simulink model "IntegratedDepthWheel"  (R2024a)
settings: Solver=VariableStepAuto  StartTime=0.0  StopTime=100  FixedStep=0.01  MaxStep=0.01  RelTol=1e-6
model workspace (MAT data in the model file):
  E_A = 10000000
  L0_init = 100
  Lambda_eff_g = 7.85
  r_wheel = 0.0508
  rho_mud = 1200
  w_tool_g = 2943
libraries: fl_lib x24, nesl_utility x9, sdl_lib x1
settings Model: Creator=Youssef  LastModifiedBy=Youssef

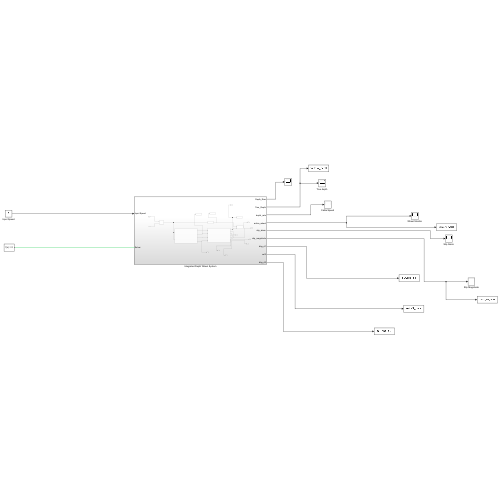
[thumbnail: Simulink's stored preview of the top-level diagram]
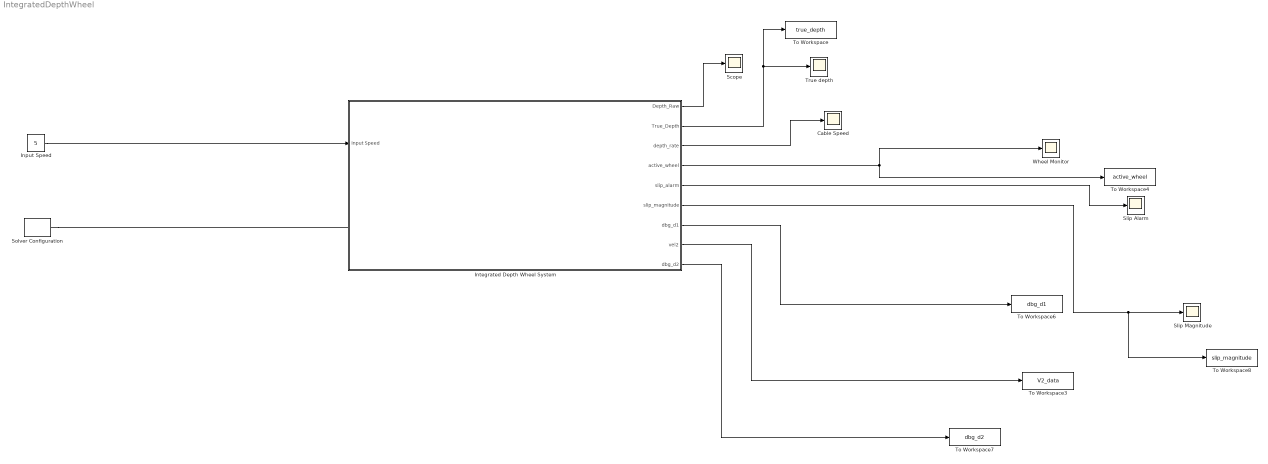
== system IntegratedDepthWheel ==
  Cable Speed : Scope
  Input Speed : Constant  Value=5
  Integrated Depth Wheel System : Subsystem
  Scope : Scope
  Slip Alarm : Scope
  Slip Magnitude : Scope
  Solver Configuration : nesl_utility/Solver Configuration  PhysicalDomain=network_engine_domain  SubClassName=solver  LeftPortType=input  RightPortType=generic  Tones=[]  Harmonics=[]  SimulateNoise=off  Profile=off  UseLocalSampling=off  EnableSwitchedLinearOptims=on  FrequencyDomain=off  UseCCode=off  RelTol=0.001  AbsTol=0.001  MinStep=1e-09  ToWorkspace=off  RevertToSquareIcSolve=off  NumHomotopyIterations=100  PhasorMode=off  PhasorModeNumHarmonics=1  ConsistencySolver=NEWTON_XTOL_AFTER_FTOL  IndexReductionMethod=DerivativeReplacement  DoDC=off  ResidualTolerance=1e-09  ConsistencyTolSource=GLOBAL  ConsistencyAbsTol=0.001  ConsistencyRelTol=0.001  ConsistencyTolFactor=0.001  UseLocalSolver=on  LocalSolverChoice=NE_TRAPEZOIDAL_ADVANCER  ResolveIndetEquations=on  FunctionEvalNumThread=1  LocalSolverSampleTime=0.01  DoFixedCost=on  MaxNonlinIter=3  MaxModeIter=2  ComputeImpulses=off  ImpulseIterations=2  LinearAlgebra=auto  LinearAlgebraNumThread=0  EquationFormulation=NE_TIME_EF  DelaysMemoryBudget=1024  AutomaticFiltering=on  FilteringTimeConstant=0.001  PartitionStorageMethod=AS_NEEDED  PartitionMemoryBudget=1024  PartitionMethod=ROBUST  MultibodyUseLocalSolver=off  MultibodyLocalSolverChoice=ODE1  MultibodyLocalSolverSampleTime=0.001
  To Workspace : ToWorkspace  VariableName=true_depth  SaveFormat=Timeseries  SampleTime=-1
  To Workspace3 : ToWorkspace  VariableName=V2_data  SaveFormat=Timeseries  SampleTime=-1
  To Workspace4 : ToWorkspace  VariableName=active_wheel  SaveFormat=Timeseries  SampleTime=-1
  To Workspace6 : ToWorkspace  VariableName=dbg_d1  SaveFormat=Timeseries  SampleTime=-1
  To Workspace7 : ToWorkspace  VariableName=dbg_d2  SaveFormat=Timeseries  SampleTime=-1
  To Workspace8 : ToWorkspace  VariableName=slip_magnitude  SaveFormat=Timeseries  SampleTime=-1
  True depth : Scope
  Wheel Monitor : Scope
  wires:
  Integrated Depth Wheel System/4(active_wheel) -> Wheel Monitor/1, To Workspace4/1
  Integrated Depth Wheel System/6(slip_magnitude) -> To Workspace8/1, Slip Magnitude/1
  Integrated Depth Wheel System/2(True_Depth) -> To Workspace/1, True depth/1
  Input Speed/1 -> Integrated Depth Wheel System/1(Input Speed)
  Integrated Depth Wheel System/1(Depth_Raw) -> Scope/1
  Integrated Depth Wheel System/3(depth_rate) -> Cable Speed/1
  Integrated Depth Wheel System/5(slip_alarm) -> Slip Alarm/1
  Integrated Depth Wheel System/7(dbg_d1) -> To Workspace6/1
  Integrated Depth Wheel System/8(vel2) -> To Workspace3/1
  Integrated Depth Wheel System/9(dbg_d2) -> To Workspace7/1
  connections:
  Solver Configuration/RConn1 -- Integrated Depth Wheel System/LConn1

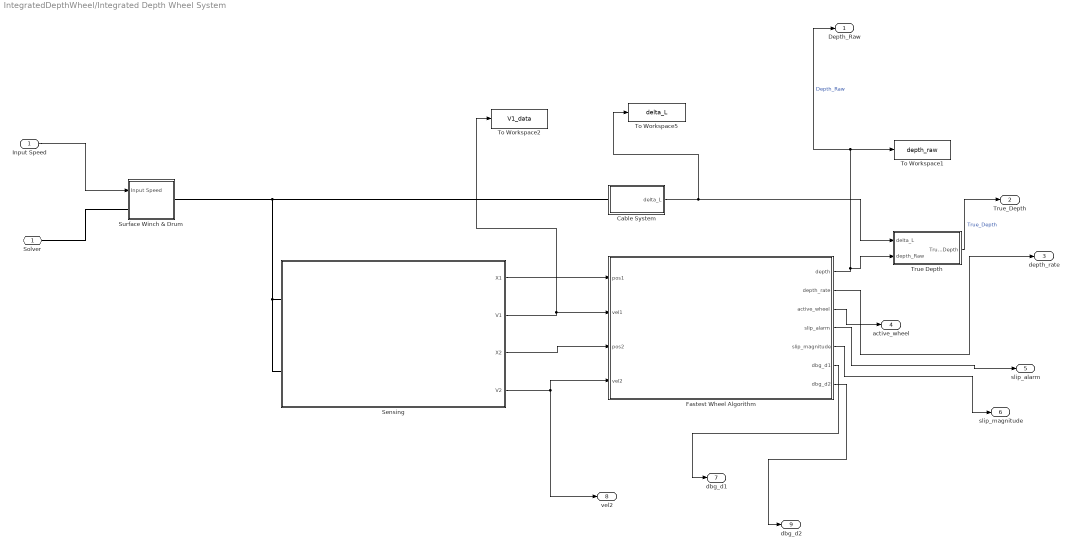
== system IntegratedDepthWheel/Integrated Depth Wheel System ==
  Input Speed : Inport
  Cable System : Subsystem
  Fastest Wheel Algorithm : MATLAB Function  TreatAsAtomicUnit=on  SystemSampleTime=0.01
  Sensing : Subsystem
  Surface Winch & Drum : Subsystem
  To Workspace1 : ToWorkspace  VariableName=depth_raw  SaveFormat=Timeseries  SampleTime=-1
  To Workspace2 : ToWorkspace  VariableName=V1_data  SaveFormat=Timeseries  SampleTime=-1
  To Workspace5 : ToWorkspace  VariableName=delta_L  SaveFormat=Timeseries  SampleTime=-1
  True Depth : Subsystem
  Solver : PMIOPort  Side=Left
  Depth_Raw : Outport
  True_Depth : Outport  Port=2
  depth_rate : Outport  Port=3
  active_wheel : Outport  Port=4
  slip_alarm : Outport  Port=5
  slip_magnitude : Outport  Port=6
  dbg_d1 : Outport  Port=7
  vel2 : Outport  Port=8
  dbg_d2 : Outport  Port=9
  wires:
  Cable System/1(delta_L) -> To Workspace5/1, True Depth/1(delta_L)
  Fastest Wheel Algorithm/1(depth) -> Depth_Raw/1, To Workspace1/1, True Depth/2(depth_Raw)  "Depth_Raw"
  Sensing/2(V1) -> To Workspace2/1, Fastest Wheel Algorithm/2(vel1)
  Sensing/4(V2) -> vel2/1, Fastest Wheel Algorithm/4(vel2)
  Sensing/3(X2) -> Fastest Wheel Algorithm/3(pos2)
  Input Speed/1 -> Surface Winch & Drum/1(Input Speed)
  Sensing/1(X1) -> Fastest Wheel Algorithm/1(pos1)
  True Depth/1(True Depth) -> True_Depth/1  "True_Depth"
  Fastest Wheel Algorithm/2(depth_rate) -> depth_rate/1
  Fastest Wheel Algorithm/5(slip_magnitude) -> slip_magnitude/1
  Fastest Wheel Algorithm/6(dbg_d1) -> dbg_d1/1
  Fastest Wheel Algorithm/4(slip_alarm) -> slip_alarm/1
  Fastest Wheel Algorithm/7(dbg_d2) -> dbg_d2/1
  Fastest Wheel Algorithm/3(active_wheel) -> active_wheel/1
  connections:
  Surface Winch & Drum/RConn1 -- Sensing/LConn2 -- Sensing/LConn1 -- Cable System/LConn1
  Solver/RConn1 -- Surface Winch & Drum/LConn1

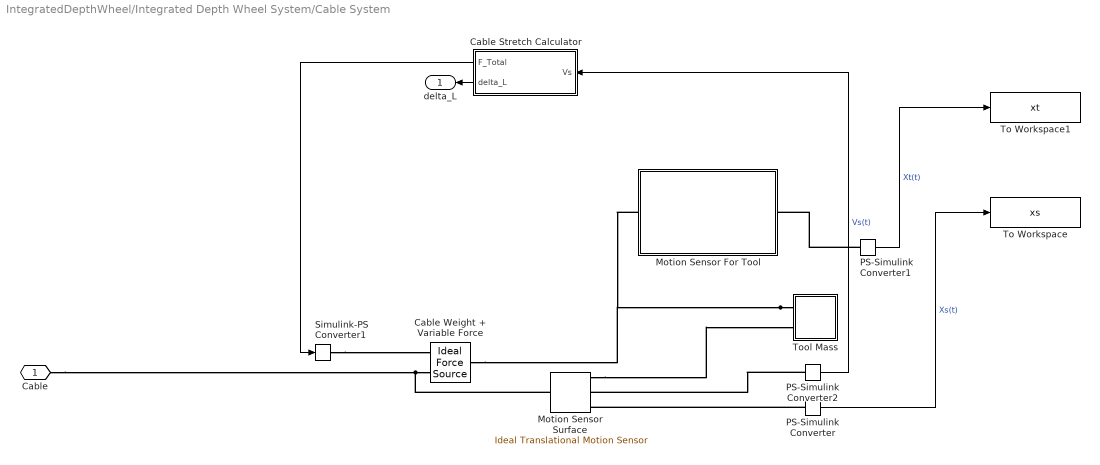
== system IntegratedDepthWheel/Integrated Depth Wheel System/Cable System ==
  " Cable Stretch Calculator" : Subsystem
  Cable Weight + Variable Force : fl_lib/Mechanical/Mechanical Sources/Ideal Force Source
  Motion Sensor For Tool : Subsystem
  Motion Sensor Surface : fl_lib/Mechanical/Mechanical Sensors/Ideal Translational Motion Sensor  reference=foundation.enum.MeasurementReference.difference  acceleration_port=false  velocity_port=true  position_port=true  offset=0 m
  PS-Simulink Converter : nesl_utility/PS-Simulink Converter  PhysicalDomain=network_engine_domain  SubClassName=ps_output  LeftPortType=input  RightPortType=output  PseudoPeriodic=off  Frequencies=[]  VectorFormat=inherit  Unit=inherit  AffineConversion=off
  PS-Simulink Converter1 : nesl_utility/PS-Simulink Converter  PhysicalDomain=network_engine_domain  SubClassName=ps_output  LeftPortType=input  RightPortType=output  PseudoPeriodic=off  Frequencies=[]  VectorFormat=inherit  Unit=inherit  AffineConversion=off
  PS-Simulink Converter2 : nesl_utility/PS-Simulink Converter  PhysicalDomain=network_engine_domain  SubClassName=ps_output  LeftPortType=input  RightPortType=output  PseudoPeriodic=off  Frequencies=[]  VectorFormat=inherit  Unit=inherit  AffineConversion=off
  Simulink-PS Converter1 : nesl_utility/Simulink-PS Converter  PhysicalDomain=network_engine_domain  SubClassName=ps_input  LeftPortType=input  RightPortType=output  PseudoPeriodic=off  Frequencies=[]  NoiseDistribution=none  NoiseParameters=[]  Unit=1  AffineConversion=off  FilteringAndDerivatives=filter  SimscapeFilterOrder=1  InputFilterTimeConstant=0.01  UdotUserProvided=0
  To Workspace : ToWorkspace  VariableName=xs  SaveFormat=Timeseries  SampleTime=-1
  To Workspace1 : ToWorkspace  VariableName=xt  SaveFormat=Timeseries  SampleTime=-1
  Tool Mass : Subsystem
  Cable : PMIOPort  Side=Left
  delta_L : Outport
  wires:
  " Cable Stretch Calculator"/2(delta_L) -> delta_L/1
  PS-Simulink Converter1/1 -> To Workspace1/1  "Xt(t)"
  " Cable Stretch Calculator"/1(F_Total) -> Simulink-PS Converter1/1
  PS-Simulink Converter/1 -> To Workspace/1  "Xs(t)"
  PS-Simulink Converter2/1 -> " Cable Stretch Calculator"/1(Vs)  "Vs(t)"
  connections:
  PS-Simulink Converter1/LConn1 -- Motion Sensor For Tool/RConn1
  Simulink-PS Converter1/RConn1 -- Cable Weight + Variable Force/RConn1
  Motion Sensor Surface/RConn1 -- Tool Mass/LConn2
  PS-Simulink Converter/LConn1 -- Motion Sensor Surface/RConn3
  Motion Sensor Surface/LConn1 -- Cable/RConn1 -- Cable Weight + Variable Force/RConn2
  Tool Mass/LConn1 -- Cable Weight + Variable Force/LConn1 -- Motion Sensor For Tool/LConn1
  PS-Simulink Converter2/LConn1 -- Motion Sensor Surface/RConn2

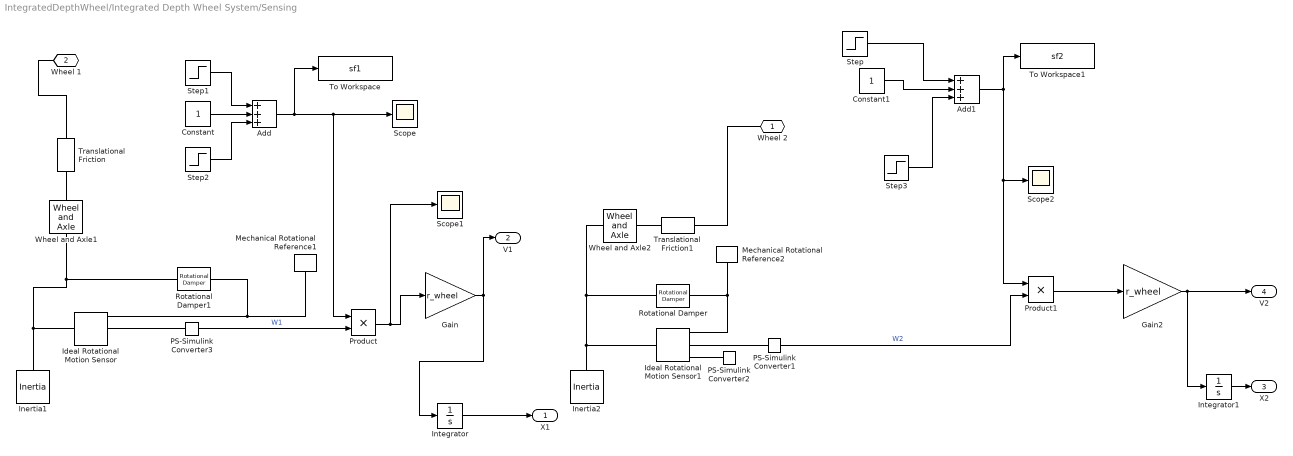
== system IntegratedDepthWheel/Integrated Depth Wheel System/Sensing ==
  Add : Sum  Inputs=+++
  Add1 : Sum  Inputs=+++
  Constant : Constant
  Constant1 : Constant
  Gain : Gain  Gain=r_wheel
  Gain2 : Gain  Gain=r_wheel
  Ideal Rotational Motion Sensor : fl_lib/Mechanical/Mechanical Sensors/Ideal Rotational Motion Sensor  reference=foundation.enum.MeasurementReference.difference  acceleration_port=false  velocity_port=true  position_port=true  wrap_angle=false  offset=0 rad
  Ideal Rotational Motion Sensor1 : fl_lib/Mechanical/Mechanical Sensors/Ideal Rotational Motion Sensor  reference=foundation.enum.MeasurementReference.difference  acceleration_port=false  velocity_port=true  position_port=true  wrap_angle=false  offset=0 rad
  Inertia1 : fl_lib/Mechanical/Rotational Elements/Inertia  inertia=0.02 kg*m^2  num_ports=foundation.enum.numPorts2.one  w_specify=off  w_priority=High  w=0 rad/s  w_nominal_specify=off  w_nominal_value=1  w_nominal_unit=rad/s  t_specify=off  t_priority=None  t=0 N*m  t_nominal_specify=off  t_nominal_value=1  t_nominal_unit=N*m
  Inertia2 : fl_lib/Mechanical/Rotational Elements/Inertia  inertia=0.02 kg*m^2  num_ports=foundation.enum.numPorts2.one  w_specify=off  w_priority=High  w=0 rad/s  w_nominal_specify=off  w_nominal_value=1  w_nominal_unit=rad/s  t_specify=off  t_priority=None  t=0 N*m  t_nominal_specify=off  t_nominal_value=1  t_nominal_unit=N*m
  Integrator : Integrator
  Integrator1 : Integrator
  Mechanical Rotational Reference1 : fl_lib/Mechanical/Rotational Elements/Mechanical Rotational Reference
  Mechanical Rotational Reference2 : fl_lib/Mechanical/Rotational Elements/Mechanical Rotational Reference
  PS-Simulink Converter1 : nesl_utility/PS-Simulink Converter  PhysicalDomain=network_engine_domain  SubClassName=ps_output  LeftPortType=input  RightPortType=output  PseudoPeriodic=off  Frequencies=[]  VectorFormat=inherit  Unit=inherit  AffineConversion=off
  PS-Simulink Converter2 : nesl_utility/PS-Simulink Converter  PhysicalDomain=network_engine_domain  SubClassName=ps_output  LeftPortType=input  RightPortType=output  PseudoPeriodic=off  Frequencies=[]  VectorFormat=inherit  Unit=inherit  AffineConversion=off
  PS-Simulink Converter3 : nesl_utility/PS-Simulink Converter  PhysicalDomain=network_engine_domain  SubClassName=ps_output  LeftPortType=input  RightPortType=output  PseudoPeriodic=off  Frequencies=[]  VectorFormat=inherit  Unit=inherit  AffineConversion=off
  Product : Product
  Product1 : Product
  Rotational Damper : fl_lib/Mechanical/Rotational Elements/Rotational Damper  D=0.001 N*m*s/rad  w_specify=off  w_priority=None  w=0 rad/s  w_nominal_specify=off  w_nominal_value=1  w_nominal_unit=rad/s  t_specify=off  t_priority=None  t=0 N*m  t_nominal_specify=off  t_nominal_value=1  t_nominal_unit=N*m
  Rotational Damper1 : fl_lib/Mechanical/Rotational Elements/Rotational Damper  D=0.001 N*m*s/rad  w_specify=off  w_priority=None  w=0 rad/s  w_nominal_specify=off  w_nominal_value=1  w_nominal_unit=rad/s  t_specify=off  t_priority=None  t=0 N*m  t_nominal_specify=off  t_nominal_value=1  t_nominal_unit=N*m
  Scope : Scope
  Scope1 : Scope
  Scope2 : Scope
  Step : Step  Time=55  After=-0.4  SampleTime=0
  Step1 : Step  Time=35  After=-0.2  SampleTime=0
  Step2 : Step  Time=50  After=0.2  SampleTime=0
  Step3 : Step  Time=70  After=0.4  SampleTime=0
  To Workspace : ToWorkspace  VariableName=sf1  SaveFormat=Timeseries  SampleTime=-1
  To Workspace1 : ToWorkspace  VariableName=sf2  SaveFormat=Timeseries  SampleTime=-1
  Translational Friction : fl_lib/Mechanical/Translational Elements/Translational Friction  brkwy_frc=100 N  brkwy_vel=0.1 m/s  Col_frc=20 N  visc_coef=100 N*s/m  v_specify=off  v_priority=None  v=0 m/s  v_nominal_specify=off  v_nominal_value=1  v_nominal_unit=m/s  f_specify=off  f_priority=None  f=0 N  f_nominal_specify=off  f_nominal_value=1  f_nominal_unit=N
      settings: InternalSimscapePortConfiguration="{\"Bottom\":[],\"Left\":[{\"id\":\"R\",\"label\":\"R\",\"type\":\"foundation.mechanical.translational.translational\"}],\"Right\":[{\"id\":\"C\",\"label\":\"C\",\"type\":\"foundation.mechanical.translational.translational\"}],\"Top\":[]}"
  Translational Friction1 : fl_lib/Mechanical/Translational Elements/Translational Friction  brkwy_frc=90 N  brkwy_vel=0.1 m/s  Col_frc=20 N  visc_coef=100 N*s/m  v_specify=off  v_priority=None  v=0 m/s  v_nominal_specify=off  v_nominal_value=1  v_nominal_unit=m/s  f_specify=off  f_priority=None  f=0 N  f_nominal_specify=off  f_nominal_value=1  f_nominal_unit=N
      settings: InternalSimscapePortConfiguration="{\"Bottom\":[],\"Left\":[{\"id\":\"R\",\"label\":\"R\",\"type\":\"foundation.mechanical.translational.translational\"}],\"Right\":[{\"id\":\"C\",\"label\":\"C\",\"type\":\"foundation.mechanical.translational.translational\"}],\"Top\":[]}"
  Wheel and Axle1 : fl_lib/Mechanical/Mechanisms/Wheel and Axle  R=r_wheel m  or=1  t_specify=off  t_priority=None  t=0 N*m  t_nominal_specify=off  t_nominal_value=1  t_nominal_unit=N*m  f_specify=off  f_priority=None  f=0 N  f_nominal_specify=off  f_nominal_value=1  f_nominal_unit=N
  Wheel and Axle2 : fl_lib/Mechanical/Mechanisms/Wheel and Axle  R=r_wheel m  or=1  t_specify=off  t_priority=None  t=0 N*m  t_nominal_specify=off  t_nominal_value=1  t_nominal_unit=N*m  f_specify=off  f_priority=None  f=0 N  f_nominal_specify=off  f_nominal_value=1  f_nominal_unit=N
  Wheel 2 : PMIOPort  Side=Left
  Wheel 1 : PMIOPort  Port=2  Side=Left
  X1 : Outport
  V1 : Outport  Port=2
  X2 : Outport  Port=3
  V2 : Outport  Port=4
  wires:
  PS-Simulink Converter3/1 -> Product/2  "W1"
  Gain/1 -> Integrator/1, V1/1
  Gain2/1 -> V2/1, Integrator1/1
  Add/1 -> To Workspace/1, Product/1, Scope/1
  Product/1 -> Scope1/1, Gain/1
  Product1/1 -> Gain2/1
  PS-Simulink Converter1/1 -> Product1/2  "W2"
  Integrator/1 -> X1/1
  Integrator1/1 -> X2/1
  Add1/1 -> To Workspace1/1, Scope2/1, Product1/1
  Step1/1 -> Add/1
  Step2/1 -> Add/3
  Constant/1 -> Add/2
  Step/1 -> Add1/1
  Constant1/1 -> Add1/2
  Step3/1 -> Add1/3
  connections:
  Inertia1/LConn1 -- Ideal Rotational Motion Sensor/LConn1 -- Rotational Damper1/LConn1 -- Wheel and Axle1/LConn1
  Inertia2/LConn1 -- Ideal Rotational Motion Sensor1/LConn1 -- Wheel and Axle2/LConn1 -- Rotational Damper/LConn1
  Translational Friction1/LConn1 -- Wheel and Axle2/RConn1
  Ideal Rotational Motion Sensor/RConn1 -- Rotational Damper1/RConn1 -- Mechanical Rotational Reference1/LConn1
  Wheel and Axle1/RConn1 -- Translational Friction/LConn1
  Translational Friction/RConn1 -- Wheel 1/RConn1
  Translational Friction1/RConn1 -- Wheel 2/RConn1
  PS-Simulink Converter3/LConn1 -- Ideal Rotational Motion Sensor/RConn2
  Ideal Rotational Motion Sensor1/RConn1 -- Mechanical Rotational Reference2/LConn1 -- Rotational Damper/RConn1
  PS-Simulink Converter1/LConn1 -- Ideal Rotational Motion Sensor1/RConn2
  PS-Simulink Converter2/LConn1 -- Ideal Rotational Motion Sensor1/RConn3

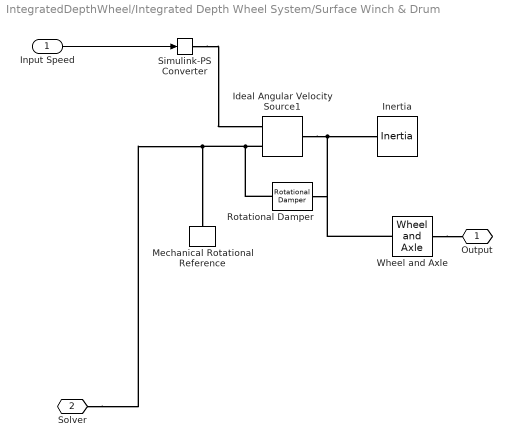
== system IntegratedDepthWheel/Integrated Depth Wheel System/Surface Winch & Drum ==
  Input Speed : Inport
  Ideal Angular Velocity Source1 : fl_lib/Mechanical/Mechanical Sources/Ideal Angular Velocity Source
  Inertia : fl_lib/Mechanical/Rotational Elements/Inertia  inertia=500 kg*m^2  num_ports=foundation.enum.numPorts2.one  w_specify=off  w_priority=High  w=0 rad/s  w_nominal_specify=off  w_nominal_value=1  w_nominal_unit=rad/s  t_specify=off  t_priority=None  t=0 N*m  t_nominal_specify=off  t_nominal_value=1  t_nominal_unit=N*m
  Mechanical Rotational Reference : fl_lib/Mechanical/Rotational Elements/Mechanical Rotational Reference
  Rotational Damper : fl_lib/Mechanical/Rotational Elements/Rotational Damper  D=0.001 N*m*s/rad  w_specify=off  w_priority=None  w=0 rad/s  w_nominal_specify=off  w_nominal_value=1  w_nominal_unit=rad/s  t_specify=off  t_priority=None  t=0 N*m  t_nominal_specify=off  t_nominal_value=1  t_nominal_unit=N*m
  Simulink-PS Converter : nesl_utility/Simulink-PS Converter  PhysicalDomain=network_engine_domain  SubClassName=ps_input  LeftPortType=input  RightPortType=output  PseudoPeriodic=off  Frequencies=[]  NoiseDistribution=none  NoiseParameters=[]  Unit=1  AffineConversion=off  FilteringAndDerivatives=provide  SimscapeFilterOrder=1  InputFilterTimeConstant=0.001  UdotUserProvided=0
  Wheel and Axle : fl_lib/Mechanical/Mechanisms/Wheel and Axle  R=0.4 m  or=1  t_specify=off  t_priority=None  t=0 N*m  t_nominal_specify=off  t_nominal_value=1  t_nominal_unit=N*m  f_specify=off  f_priority=None  f=0 N  f_nominal_specify=off  f_nominal_value=1  f_nominal_unit=N
  Output : PMIOPort  Side=Right
  Solver : PMIOPort  Port=2  Side=Left
  wires:
  Input Speed/1 -> Simulink-PS Converter/1
  connections:
  Ideal Angular Velocity Source1/RConn2 -- Rotational Damper/RConn1 -- Solver/RConn1 -- Mechanical Rotational Reference/LConn1
  Ideal Angular Velocity Source1/LConn1 -- Wheel and Axle/LConn1 -- Rotational Damper/LConn1 -- Inertia/LConn1
  Simulink-PS Converter/RConn1 -- Ideal Angular Velocity Source1/RConn1
  Wheel and Axle/RConn1 -- Output/RConn1

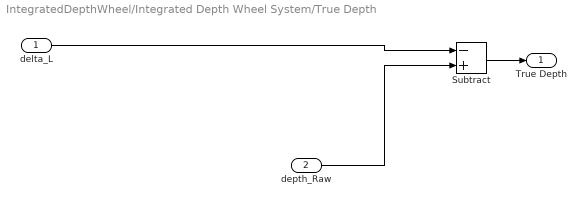
== system IntegratedDepthWheel/Integrated Depth Wheel System/True Depth ==
  delta_L : Inport
  depth_Raw : Inport  Port=2
  Subtract : Sum  Inputs=-+
  True Depth : Outport
  wires:
  delta_L/1 -> Subtract/1
  depth_Raw/1 -> Subtract/2
  Subtract/1 -> True Depth/1

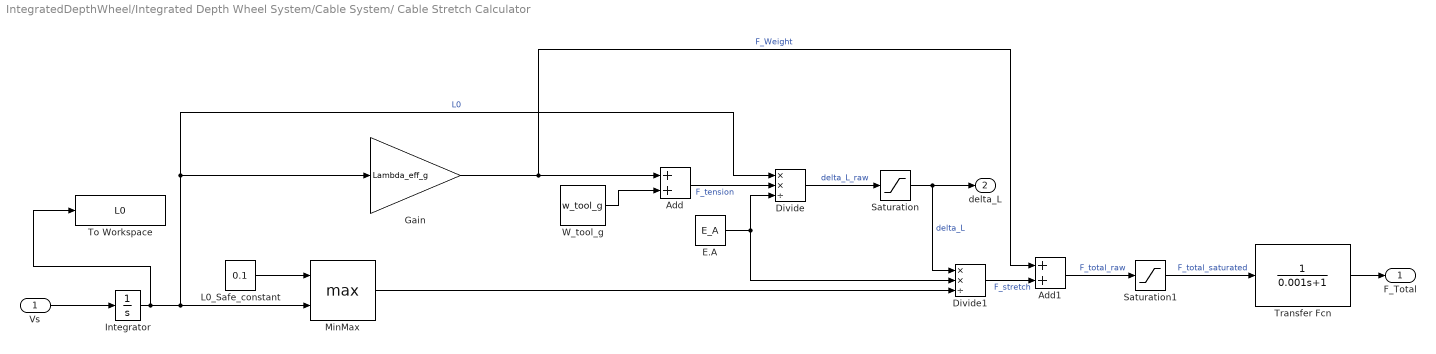
== system IntegratedDepthWheel/Integrated Depth Wheel System/Cable System/ Cable Stretch Calculator ==
  Vs : Inport
  Add : Sum
  Add1 : Sum
  Divide : Product  Inputs=**/
  Divide1 : Product  Inputs=**/
  E.A : Constant  Value=E_A
  Gain : Gain  Gain=Lambda_eff_g
  Integrator : Integrator  InitialCondition=L0_init
  L0_Safe_constant : Constant  Value=0.1
  MinMax : MinMax  Function=max  Inputs=2
  Saturation : Saturate  UpperLimit=inf  LowerLimit=0
  Saturation1 : Saturate  UpperLimit=50000  LowerLimit=0
  To Workspace : ToWorkspace  VariableName=L0  SaveFormat=Timeseries  SampleTime=-1
  Transfer Fcn : TransferFcn  Denominator=[0.001 1]
  W_tool_g : Constant  Value=w_tool_g
  F_Total : Outport
  delta_L : Outport  Port=2
  wires:
  Vs/1 -> Integrator/1
  Integrator/1 -> To Workspace/1, Divide/1, Gain/1, MinMax/2  "L0"
  L0_Safe_constant/1 -> MinMax/1
  Gain/1 -> Add1/1, Add/1  "F_Weight"
  W_tool_g/1 -> Add/2
  Add/1 -> Divide/2  "F_tension"
  E.A/1 -> Divide1/2, Divide/3
  Divide/1 -> Saturation/1  "delta_L_raw"
  Saturation/1 -> Divide1/1, delta_L/1  "delta_L"
  MinMax/1 -> Divide1/3
  Divide1/1 -> Add1/2  "F_stretch"
  Add1/1 -> Saturation1/1  "F_total_raw"
  Saturation1/1 -> Transfer Fcn/1  "F_total_saturated"
  Transfer Fcn/1 -> F_Total/1

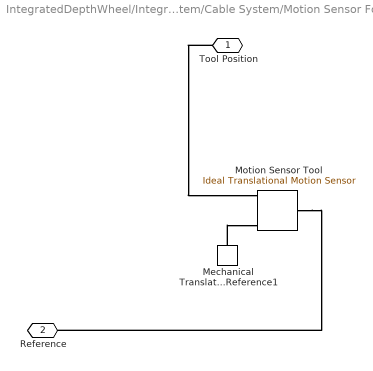
== system IntegratedDepthWheel/Integrated Depth Wheel System/Cable System/Motion Sensor For Tool ==
  Mechanical Translational Reference1 : fl_lib/Mechanical/Translational Elements/Mechanical Translational Reference
  Motion Sensor Tool : fl_lib/Mechanical/Mechanical Sensors/Ideal Translational Motion Sensor  reference=foundation.enum.MeasurementReference.difference  acceleration_port=false  velocity_port=true  position_port=true  offset=0 m
  Tool Position : PMIOPort  Side=Right
  Reference : PMIOPort  Port=2  Side=Left
  connections:
  Motion Sensor Tool/LConn1 -- Reference/RConn1
  Mechanical Translational Reference1/LConn1 -- Motion Sensor Tool/RConn1
  Tool Position/RConn1 -- Motion Sensor Tool/RConn3

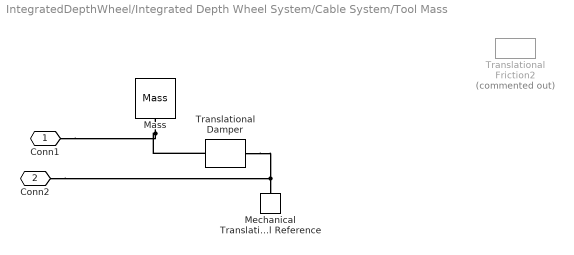
== system IntegratedDepthWheel/Integrated Depth Wheel System/Cable System/Tool Mass ==
  Mass : fl_lib/Mechanical/Translational Elements/Mass  mass=500 kg  num_ports=foundation.enum.numPorts2.one  v_specify=off  v_priority=High  v=0 m/s  v_nominal_specify=off  v_nominal_value=1  v_nominal_unit=m/s  f_specify=off  f_priority=None  f=0 N  f_nominal_specify=off  f_nominal_value=1  f_nominal_unit=N
  Mechanical Translational Reference : fl_lib/Mechanical/Translational Elements/Mechanical Translational Reference
  Translational Friction2 : fl_lib/Mechanical/Translational Elements/Translational Friction  Commented=on  brkwy_frc=90 N  brkwy_vel=0.1 m/s  Col_frc=20 N  visc_coef=100 N*s/m  v_specify=off  v_priority=None  v=0 m/s  v_nominal_specify=off  v_nominal_value=1  v_nominal_unit=m/s  f_specify=off  f_priority=None  f=0 N  f_nominal_specify=off  f_nominal_value=1  f_nominal_unit=N
      settings: InternalSimscapePortConfiguration="{\"Bottom\":[],\"Left\":[{\"id\":\"R\",\"label\":\"R\",\"type\":\"foundation.mechanical.translational.translational\"}],\"Right\":[{\"id\":\"C\",\"label\":\"C\",\"type\":\"foundation.mechanical.translational.translational\"}],\"Top\":[]}"
  Translational Damper : sdl_lib/Couplings & Drives/Springs & Dampers/Translational Damper  D=100 N*s/m  enable_faults=simscape.enum.onoff.off  b_fault=1e6 N*s/m  fault_trigger=simscape.fault.triggertype.external  acceleration_limit=100 m/s^2  shock_limit=1  thermal_port=simscape.enum.thermaleffects.omit  thermal_mass=50 kJ/K  temperature_specify=off  temperature_priority=High  temperature=300 K  temperature_nominal_specify=off  temperature_nominal_value=1  temperature_nominal_unit=K
  Conn1 : PMIOPort  Side=Left
  Conn2 : PMIOPort  Port=2  Side=Left
  connections:
  Mechanical Translational Reference/LConn1 -- Translational Damper/RConn1 -- Conn2/RConn1
  Mass/LConn1 -- Translational Damper/LConn1 -- Conn1/RConn1

== matlab function IntegratedDepthWheel/Integrated Depth Wheel System/Fastest Wheel Algorithm ==
  data: pos1 input; depth output; vel1 input; pos2 input; vel2 input; depth_rate output; active_wheel output; slip_alarm output; slip_magnitude output; dbg_d1 output; dbg_d2 output
function [depth, depth_rate, active_wheel, slip_alarm, slip_magnitude, dbg_d1, dbg_d2] = ...
         fastest_wheel(pos1, vel1, pos2, vel2)
%==========================================================================
% FASTEST WHEEL DEPTH ACQUISITION ALGORITHM
% Schlumberger Patent US4924596 / Halliburton WSDP AMS4A043
%==========================================================================

%--------------------------------------------------------------------------
% PARAMETERS
%--------------------------------------------------------------------------
switch_threshold = 0.05;   % m/s — minimum velocity difference to switch wheel
LV               = 0.005;  % m   — slip detection threshold per sample
                            %       reduced from 0.5 inch for simulation
slip_limit       = 0.1016; % m   — cumulative slip alarm limit (4 inches)

%--------------------------------------------------------------------------
% PERSISTENT STATE
%--------------------------------------------------------------------------
persistent depth_accum
persistent pos1_prev
persistent pos2_prev
persistent slip_counter
persistent alarm_latched
persistent active_wheel_state

if isempty(depth_accum)
    depth_accum        = 0;
    pos1_prev          = pos1;
    pos2_prev          = pos2;
    slip_counter       = 0;
    alarm_latched      = 0;
    active_wheel_state = 1;
end

%--------------------------------------------------------------------------
% LAYER 1 — DELTA COMPUTATION
%--------------------------------------------------------------------------
delta1 = pos1 - pos1_prev;
delta2 = pos2 - pos2_prev;

%--------------------------------------------------------------------------
% LAYER 2 — WHEEL SELECTION
%--------------------------------------------------------------------------
vel_diff = abs(vel1) - abs(vel2);

if vel_diff > switch_threshold
    active_wheel_state = 1;
elseif vel_diff < -switch_threshold
    active_wheel_state = 2;
end

active_wheel = active_wheel_state;

if active_wheel == 1
    chosen_delta = delta1;
    depth_rate   = vel1;
else
    chosen_delta = delta2;
    depth_rate   = vel2;
end

%--------------------------------------------------------------------------
% LAYER 3 — DEPTH ACCUMULATION
%--------------------------------------------------------------------------
depth_accum = depth_accum + chosen_delta;
depth       = depth_accum;

%--------------------------------------------------------------------------
% LAYER 4 — SLIP DETECTION
% Per Schlumberger US4924596:
% Slip is registered whenever the two wheels disagree by more than LV
% This is independent of which wheel the algorithm selected
% It is a DATA QUALITY flag — tells operator a slip event occurred
% Even if depth was protected, the event is recorded
%--------------------------------------------------------------------------
delta_diff = abs(delta1 - delta2);

% Detect slip event — wheels disagreeing
wheel1_slower = abs(vel1) < abs(vel2) - switch_threshold;
wheel2_slower = abs(vel2) < abs(vel1) - switch_threshold;
slip_event    = wheel1_slower || wheel2_slower;

if slip_event && delta_diff > LV
    % Slip confirmed — accumulate magnitude
    slip_counter = slip_counter + delta_diff;
elseif ~slip_event
    % Both wheels agree — slowly decay the counter
    % Represents operator acknowledgment window
    slip_counter = max(0, slip_counter - LV * 0.1);
end

% Alarm latches when cumulative slip exceeds 4 inches
% Resets when counter decays back to zero
if slip_counter > slip_limit
    alarm_latched = 1;
elseif slip_counter <= 0
    alarm_latched = 0;
end

slip_alarm     = alarm_latched;
slip_magnitude = slip_counter;

%--------------------------------------------------------------------------
% LAYER 5 — STATE UPDATE
%--------------------------------------------------------------------------
pos1_prev = pos1;
pos2_prev = pos2;

dbg_d1 = delta1;
dbg_d2 = delta2;
